simulink model "samplModel_R2018b"  (R2018b)
settings: Solver=FixedStepDiscrete  StartTime=0.0  StopTime=10  RelTol=1e-3  EnableMultiTasking=on
settings Model: Creator=stozaki  LastModifiedBy=stozaki
settings DataIOCC: LimitDataPoints=on  SaveFormat=Array  VisualizeSimOutput=off
settings OptimizationCC: DefaultParameterBehavior=Inlined  LifeSpan=1
settings DebuggingCC: AlgebraicLoopMsg=error  ParameterDowncastMsg=warning  ParameterOverflowMsg=warning  ParameterUnderflowMsg=warning  FixptConstUnderflowMsg=warning  FixptConstOverflowMsg=warning  FixptConstPrecisionLossMsg=warning  StateNameClashWarn=warning  SFUnexpectedBacktrackingDiag=warning  SFNoUnconditionalDefaultTransitionDiag=warning  SFExecutionAtInitializationDiag=none
settings HardwareCC: ProdBitPerPointer=32  ProdBitPerSizeT=32  ProdBitPerPtrDiffT=32  ProdLargestAtomicFloat=None  ProdIntDivRoundTo=Undefined  ProdEndianess=Unspecified  ProdWordSize=32  ProdHWDeviceType=Generic->32-bit Embedded Processor  TargetHWDeviceType=Generic->Custom  ProdEqTarget=off
settings ModelReferenceCC: PropagateSignalLabelsOutOfModel=off
settings SFSimCC: SimUseLocalCustomCode=off  MATLABDynamicMemAlloc=off
settings RTWCC: SystemTargetFile=ert.tlc  TemplateMakefile=ert_default_tmf  GenerateReport=on  RTWUseLocalCustomCode=off  IncludeHyperlinkInReport=on  LaunchReport=on  GenerateCodeMetricsReport=on
settings CodeAppCC: IgnoreCustomStorageClasses=off  StateflowObjectComments=on
settings ERTTargetCC: MultiwordLength=2048  GenerateSampleERTMain=on  InlinedParameterPlacement=NonHierarchical  ERTCustomFileTemplate=example_file_process.tlc  ConvertIfToSwitch=off  SuppressUnreachableDefaultCases=off
settings ConfigComp: CovMetricSettings=dw  CovHtmlReporting=on  CovSaveCumulativeToWorkspaceVar=on  CovSaveSingleToWorkspaceVar=on  CovExternalEMLEnable=off

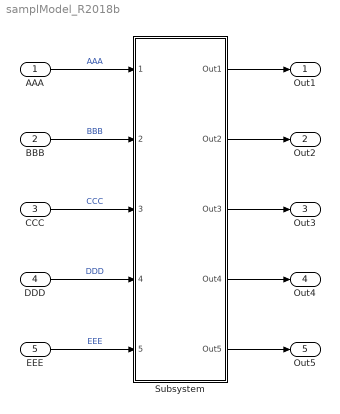
== system samplModel_R2018b ==
  AAA : Inport
  BBB : Inport  Port=2
  CCC : Inport  Port=3
  DDD : Inport  Port=4
  EEE : Inport  Port=5
  Subsystem : Subsystem
  Out1 : Outport
  Out2 : Outport  Port=2
  Out3 : Outport  Port=3
  Out4 : Outport  Port=4
  Out5 : Outport  Port=5
  wires:
  AAA/1 -> Subsystem/1(1)  "AAA"
  BBB/1 -> Subsystem/2(2)  "BBB"
  CCC/1 -> Subsystem/3(3)  "CCC"
  DDD/1 -> Subsystem/4(4)  "DDD"
  EEE/1 -> Subsystem/5(5)  "EEE"
  Subsystem/1(Out1) -> Out1/1
  Subsystem/2(Out2) -> Out2/1
  Subsystem/3(Out3) -> Out3/1
  Subsystem/4(Out4) -> Out4/1
  Subsystem/5(Out5) -> Out5/1

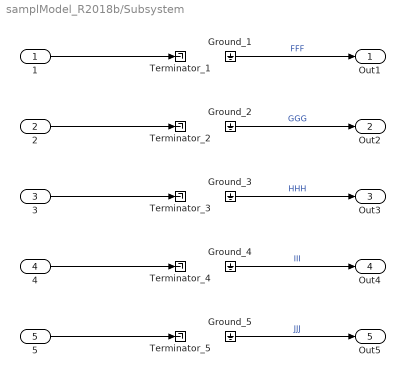
== system samplModel_R2018b/Subsystem ==
  1 : Inport
  2 : Inport  Port=2
  3 : Inport  Port=3
  4 : Inport  Port=4
  5 : Inport  Port=5
  Ground_{1..5} (5 alike) : Ground
  Terminator_{1..5} (5 alike) : Terminator
  Out1 : Outport
  Out2 : Outport  Port=2
  Out3 : Outport  Port=3
  Out4 : Outport  Port=4
  Out5 : Outport  Port=5
  wires:
  1/1 -> Terminator_1/1
  2/1 -> Terminator_2/1
  3/1 -> Terminator_3/1
  4/1 -> Terminator_4/1
  5/1 -> Terminator_5/1
  Ground_1/1 -> Out1/1  "FFF"
  Ground_2/1 -> Out2/1  "GGG"
  Ground_3/1 -> Out3/1  "HHH"
  Ground_4/1 -> Out4/1  "III"
  Ground_5/1 -> Out5/1  "JJJ"
